simulink model "open_loop"  (R2025b)
settings: Solver=VariableStepAuto  StartTime=0.0  StopTime=sim_time  RelTol=1e-3  AbsTol=1e-3  EnableMultiTasking=on
PreLoadFcn:
  | % =========================================================================
  | % CONFIGURAZIONE SPIDER-BOT: PARAMETRI UNIFICATI
  | % =========================================================================
  | clear; clc;
  | 
  | V_cmd = [0.0; 1.0; 0.0];
  | 
  | robot.L_coxa  = 0.0380;
  | robot.L_femur = 0.08625;
  | robot.L_tibia = 0.1605;
  | 
  | robot.R_hex = 0.125;
  | 
  | % NUOVO ORDINE: 1=RR, 2=RL, 3=FR, 4=FL
  | % I primi 6 output andranno alle gambe Dietro, gli ultimi 6 a quelle Davanti
  | robot.theta = [2*pi/3, -2*pi/3, pi/3, -pi/3];
  | 
  | robot.spalle_x = robot.R_hex * cos(robot.theta);
  | robot.spalle_y = robot.R_hex * sin(robot.theta);
  | robot.spalle_z = zeros(1, 4);
  | 
  | gait.step_length     = 0.060;
  | gait.step_height     = 0.035;
  | gait.cycle_duration  = 3.0;
  | gait.duty_factor     = 0.75;
  | 
  | gait.home_locale = [0.080; 0.0; -0.120];
  | 
  | sim_time = 30;
  | sim_ts = 0.01;
StartFcn:
  | % =========================================================================
  | % CONFIGURAZIONE SPIDER-BOT: PARAMETRI UNIFICATI
  | % =========================================================================
  | clear; clc;
  | 
  | V_cmd = [0.0; 1.0; 0.0];
  | 
  | robot.L_coxa  = 0.030;
  | robot.L_femur = 0.085;
  | robot.L_tibia = 0.113;
  | 
  | robot.R_hex = 0.125;
  | 
  | % NUOVO ORDINE: 1=RL, 2=RR, 3=FL, 4=FR
  | % I primi 6 output andranno alle gambe Dietro, gli ultimi 6 a quelle Davanti
  | robot.theta = [-2*pi/3, 2*pi/3, -pi/3, pi/3];
  | 
  | robot.spalle_x = robot.R_hex * cos(robot.theta);
  | robot.spalle_y = robot.R_hex * sin(robot.theta);
  | robot.spalle_z = zeros(1, 4);
  | 
  | gait.step_length     = 0.060;
  | gait.step_height     = 0.035;
  | gait.cycle_duration  = 2.0;
  | gait.duty_factor     = 0.75;
  | 
  | gait.home_locale = [0.080; 0.0; -0.120];
  | 
  | sim_time = 30;
  | sim_ts = 0.01;
undefined symbols (not defined in the file or in its folder): X, Y, Z
libraries: sm_lib x141, nesl_utility x41
(part 4 of 4)

== matlab function open_loop/MATLAB Function ==
  data: P_globali input; q_joints output; robot parameter
function q_joints = global_inverse_kinematics(P_globali, robot)
    q_joints = zeros(12, 1);
    
    Lc = robot.L_coxa;
    Lf = robot.L_femur;
    Lt = robot.L_tibia;
    
    idx = 1;
    for i = 1:4
        dx = P_globali(1, i) - robot.spalle_x(i);
        dy = P_globali(2, i) - robot.spalle_y(i);
        
        % FIX 1: The Z-coordinate MUST be relative to the shoulder joint!
        % Based on your URDF, the coxa/shoulder is at Z = 0.02.
        % If robot.spalle_z does not exist, we default to 0.02.
        if isfield(robot, 'spalle_z')
            dz = P_globali(3, i) - robot.spalle_z(i);
        else
            dz = P_globali(3, i) - 0.02; 
        end
        
        % Rotate foot target into the leg's local 2D plane
        c = cos(-robot.theta(i));
        s = sin(-robot.theta(i));
        
        loc_x = dx * c - dy * s;
        loc_y = dx * s + dy * c;
        loc_z = dz; 
        
        % 1. YAW (Coxa)
        q1 = atan2(loc_y, loc_x); 
        
        % Distance from coxa to foot in XY plane
        L_xy = sqrt(loc_x^2 + loc_y^2);
        
        % Horizontal distance for the 2D Femur/Tibia triangle
        L_forward = L_xy - Lc; 
        
        % Prevent L_forward from going negative (which causes violent leg spinning)
        if L_forward < 0
            L_forward = 0.001; 
        end
        
        % Direct hypotenuse distance from Femur joint to Foot
        D = sqrt(L_forward^2 + loc_z^2);
        
        % Clamp to prevent mathematical complex numbers (NaN) if reach is too far
        max_reach = Lf + Lt - 0.0001;
        min_reach = abs(Lf - Lt) + 0.0001;
        D = max(min(D, max_reach), min_reach);
        
        % 2. KNEE (Tibia)
        cos_q3 = (D^2 - Lf^2 - Lt^2) / (2 * Lf * Lt);
        cos_q3 = max(min(cos_q3, 1.0), -1.0); 
        
        % FIX 3: THE KNEE DIRECTION TOGGLE
        % For spiders, the knee usually bends UP. 
        % If the legs bend backwards into the ground, change this to: q3 = -acos(cos_q3);
        q3 = acos(cos_q3); 
        
        % 3. SHOULDER PITCH (Femur)
        alpha = atan2(loc_z, L_forward);
        beta  = atan2(Lt * sin(q3), Lf + Lt * cos(q3));
        q2 = alpha + beta; 
        
        % --- APPLY URDF CALIBRATION OFFSETS ---
        q_joints(idx) = q1;
        
        % FIX 2: Fixed the pi/3 (60 deg) typo to match your comment's intent (90 deg).
        % Adjust these ONLY if the robot stands perfectly but is tilted or too low.
        femur_offset_rad = pi/2; % 90 degrees
        tibia_offset_rad = pi;   % 180 degrees
        
        q_joints(idx+1) = q2 - femur_offset_rad;  
        q_joints(idx+2) = q3 - tibia_offset_rad;    
        
        idx = idx + 3;
    end
end

== matlab function open_loop/MATLAB Function2 ==
  data: t input; P_globali output; V_cmd parameter; robot parameter; gait parameter
function P_globali = trot_gait_planner(t, V_cmd, robot, gait)
    P_globali = zeros(3, 4);
    
    dir_x = 1.0;
    dir_y = 0.0;
    rot_z = 0.0;
    
    norm_v = norm([dir_x, dir_y]);
    if norm_v > 0.001
        dir_x = dir_x / norm_v;
        dir_y = dir_y / norm_v;
    else
        dir_x = 0; dir_y = 0;
    end
    
    step_length = gait.step_length;
    
    % Altezza dinamica per compensazione rollio
    step_height = gait.step_height;
    if abs(dir_y) > 0.5 
        step_height = step_height * 1.5; 
    end
    
    % Penetrazione per trazione in Simscape
    stance_depth = -0.005; 
    
    max_rot_rad = 15.0 * (pi / 180.0); 
    
    T = 0.6;
    phase_globale = (t / T) - floor(t / T);
    
    % --- NUOVA LOGICA: Offsets per andatura TROT ---
    % Sincronizzazione Diagonale. Ordine array: [RL, RR, FL, FR]
    % FL(3) e RR(2) partono a 0.0
    % FR(4) e RL(1) partono a 0.5 (mezzo ciclo dopo)
    offsets = [0.00, 0.50,0.50, 0.00 ]; 
    
    for i = 1:4
        local_phase = phase_globale + offsets(i);
        if local_phase >= 1.0
            local_phase = local_phase - 1.0;
        end
        
        th = robot.theta(i);
        c_th = cos(th); s_th = sin(th);
        
        x_home_g = robot.spalle_x(i) + (gait.home_locale(1)*c_th - gait.home_locale(2)*s_th);
        y_home_g = robot.spalle_y(i) + (gait.home_locale(1)*s_th + gait.home_locale(2)*c_th);
        z_home_g = gait.home_locale(3);
        
        % --- NUOVA LOGICA: Duty Factor 50% ---
        if local_phase < 0.50
            % Fase di Volo (Swing) - 50% del tempo
            % Moltiplichiamo per 2.0 per mappare [0.0 - 0.5] in [0.0 - 1.0]
            swingPhase = local_phase * 2.0; 
            
            step_x = dir_x * ( (-step_length / 2.0) + (step_length * swingPhase) );
            step_y = dir_y * ( (-step_length / 2.0) + (step_length * swingPhase) );
            step_rot = rot_z * ( (-max_rot_rad / 2.0) + (max_rot_rad * swingPhase) );
            
            % La zampa sale fluidamente fino a step_height
            step_z = sin(swingPhase * pi) * step_height;
        else
            % Fase di Appoggio (Stance) - 50% del tempo
            % Mappiamo [0.5 - 1.0] in [0.0 - 1.0]
            stancePhase = (local_phase - 0.50) * 2.0; 
            
            step_x = dir_x * ( (step_length / 2.0) - (step_length * stancePhase) );
            step_y = dir_y * ( (step_length / 2.0) - (step_length * stancePhase) );
            step_rot = rot_z * ( (max_rot_rad / 2.0) - (max_rot_rad * stancePhase) );
            
            % La zampa preme contro il suolo per aggrapparsi
            step_z = stance_depth; 
        end
        
        c_rot = cos(step_rot);
        s_rot = sin(step_rot);
        rot_home_x = x_home_g * c_rot - y_home_g * s_rot;
        rot_home_y = x_home_g * s_rot + y_home_g * c_rot;
        
        P_globali(1, i) = rot_home_x + step_x;
        P_globali(2, i) = rot_home_y + step_y;
        P_globali(3, i) = z_home_g + step_z;
    end
end

== matlab function open_loop/MATLAB Function3 ==
  data: t input; P_globali output; robot parameter; gait parameter
function P_globali = creep_gait_planner(t, robot, gait)
    P_globali = zeros(3, 4);
    
    dir_x = 1.0;
    dir_y = 0.0;
    rot_z = 0.0;
    
    norm_v = norm([dir_x, dir_y]);
    if norm_v > 0.001
        dir_x = dir_x / norm_v;
        dir_y = dir_y / norm_v;
    else
        dir_x = 0; dir_y = 0;
    end
    
    step_length = gait.step_length;
    
    % --- NUOVA LOGICA: Altezza dinamica ---
    % Se ci muoviamo molto lateralmente, alziamo le gambe di più (es. 1.5x)
    % per compensare l'inclinazione del robot.
    step_height = gait.step_height;
    if abs(dir_y) > 0.5 
        step_height = step_height * 1.5; 
    end
    
    % --- NUOVA LOGICA: Grip (Penetrazione) ---
    % Spingiamo il piede 5 mm sotto lo zero durante l'appoggio per fare attrito
    stance_depth = -0.005; 
    
    max_rot_rad = 15.0 * (pi / 180.0); 
    
    T = gait.cycle_duration;
    phase_globale = (t / T) - floor(t / T);
    
    % Ordine: RL, RR, FL, FR
    offsets = [0.50, 0.00, 0.75, 0.25]; 
    
    for i = 1:4
        local_phase = phase_globale + offsets(i);
        if local_phase >= 1.0
            local_phase = local_phase - 1.0;
        end
        
        th = robot.theta(i);
        c_th = cos(th); s_th = sin(th);
        
        x_home_g = robot.spalle_x(i) + (gait.home_locale(1)*c_th - gait.home_locale(2)*s_th);
        y_home_g = robot.spalle_y(i) + (gait.home_locale(1)*s_th + gait.home_locale(2)*c_th);
        z_home_g = gait.home_locale(3);
        
        if local_phase < 0.25
            % Fase di Volo
            swingPhase = local_phase * 4.0; 
            step_x = dir_x * ( (-step_length / 2.0) + (step_length * swingPhase) );
            step_y = dir_y * ( (-step_length / 2.0) + (step_length * swingPhase) );
            step_rot = rot_z * ( (-max_rot_rad / 2.0) + (max_rot_rad * swingPhase) );
            
            % La zampa sale fluidamente fino a step_height
            step_z = sin(swingPhase * pi) * step_height;
        else
            % Fase di Appoggio
            stancePhase = (local_phase - 0.25) / 0.75; 
            step_x = dir_x * ( (step_length / 2.0) - (step_length * stancePhase) );
            step_y = dir_y * ( (step_length / 2.0) - (step_length * stancePhase) );
            step_rot = rot_z * ( (max_rot_rad / 2.0) - (max_rot_rad * stancePhase) );
            
            % La zampa preme contro il suolo per aggrapparsi
            step_z = stance_depth; 
        end
        
        c_rot = cos(step_rot);
        s_rot = sin(step_rot);
        rot_home_x = x_home_g * c_rot - y_home_g * s_rot;
        rot_home_y = x_home_g * s_rot + y_home_g * c_rot;
        
        P_globali(1, i) = rot_home_x + step_x;
        P_globali(2, i) = rot_home_y + step_y;
        P_globali(3, i) = z_home_g + step_z;
    end
end

== matlab function open_loop/MATLAB Function4 ==
  data: t input; V_cmd parameter; P_globali output; robot parameter; gait parameter
function P_globali = pace_gait_planner_advanced(t, V_cmd, robot, gait)
    P_globali = zeros(3, 4);
    
    dir_x = 1.0; dir_y = 0.0; rot_z =0.0;
    
    norm_v = norm([dir_x, dir_y]);
    if norm_v > 0.001
        dir_x = dir_x / norm_v; dir_y = dir_y / norm_v;
    else
        dir_x = 0; dir_y = 0;
    end
    
    step_length = gait.step_length;
    step_height = gait.step_height;
    stance_depth = -0.005; 
    max_rot_rad = 15.0 * (pi / 180.0); 
    
    T = 0.6; 
    phase_globale = (t / T) - floor(t / T);
    
    % --- MODIFICATION 1: VIRTUAL SWAY (Lateral Weight Shift) ---
    % Shift the body left and right by 1.5 cm.
    % When phase is 0->0.5, sin() is positive (shifting body to the Left).
    % During this time, the Right legs are swinging, so the weight is safely on the Left!
    sway_amplitude = 0.015; 
    body_sway_y = sway_amplitude * sin(phase_globale * 2 * pi);
    
    % --- MODIFICATION 2: THE BROKEN PACE (Amble) ---
    % Pure Pace is: [0.00, 0.50, 0.00, 0.50]
    % Broken Pace delays the Front legs by 10% (0.10) to smooth out the impact.
    % Order: [RR, RL, FR, FL]
    offsets = [0.00, 0.50, 0.00, 0.50]; 
    
    % --- MODIFICATION 3: DUTY FACTOR TWEAK ---
    % 0.55 means legs overlap on the ground slightly, preventing lateral tipping
    duty_factor = 0.55; 
    swing_duration = 1.0 - duty_factor; % 0.45
    
    for i = 1:4
        local_phase = phase_globale + offsets(i);
        if local_phase >= 1.0
            local_phase = local_phase - 1.0;
        end
        
        th = robot.theta(i);
        c_th = cos(th); s_th = sin(th);
        
        x_home_g = robot.spalle_x(i) + (gait.home_locale(1)*c_th - gait.home_locale(2)*s_th);
        
        % Apply the Virtual Sway to the Y-coordinate of the shoulder
        y_home_g = robot.spalle_y(i) + (gait.home_locale(1)*s_th + gait.home_locale(2)*c_th) + body_sway_y;
        
        z_home_g = gait.home_locale(3);
        
        if local_phase < swing_duration
            % --- SWING PHASE ---
            swingPhase = local_phase / swing_duration; 
            
            % Velocity Matching (Teardrop Curve)
            skewed_progress = swingPhase - 0.15 * sin(swingPhase * 2 * pi);
            
            step_x = dir_x * ( (-step_length / 2.0) + (step_length * skewed_progress) );
            step_y = dir_y * ( (-step_length / 2.0) + (step_length * skewed_progress) );
            step_rot = rot_z * ( (-max_rot_rad / 2.0) + (max_rot_rad * skewed_progress) );
            
            step_z = step_height * sin(swingPhase * pi);
        else
            % --- STANCE PHASE ---
            stancePhase = (local_phase - swing_duration) / duty_factor; 
            
            step_x = dir_x * ( (step_length / 2.0) - (step_length * stancePhase) );
            step_y = dir_y * ( (step_length / 2.0) - (step_length * stancePhase) );
            step_rot = rot_z * ( (max_rot_rad / 2.0) - (max_rot_rad * stancePhase) );
            
            step_z = stance_depth; 
        end
        
        c_rot = cos(step_rot);
        s_rot = sin(step_rot);
        rot_home_x = x_home_g * c_rot - y_home_g * s_rot;
        rot_home_y = x_home_g * s_rot + y_home_g * c_rot;
        
        P_globali(1, i) = rot_home_x + step_x;
        P_globali(2, i) = rot_home_y + step_y;
        P_globali(3, i) = z_home_g + step_z;
    end
end
